simulink model "pid_control"  (R2014a)
settings: Solver=ode45  StartTime=0.0  StopTime=100.0  RelTol=1e-3
libraries: fuzblock x1
settings Model: Creator=Gaea  LastModifiedBy=Gaea

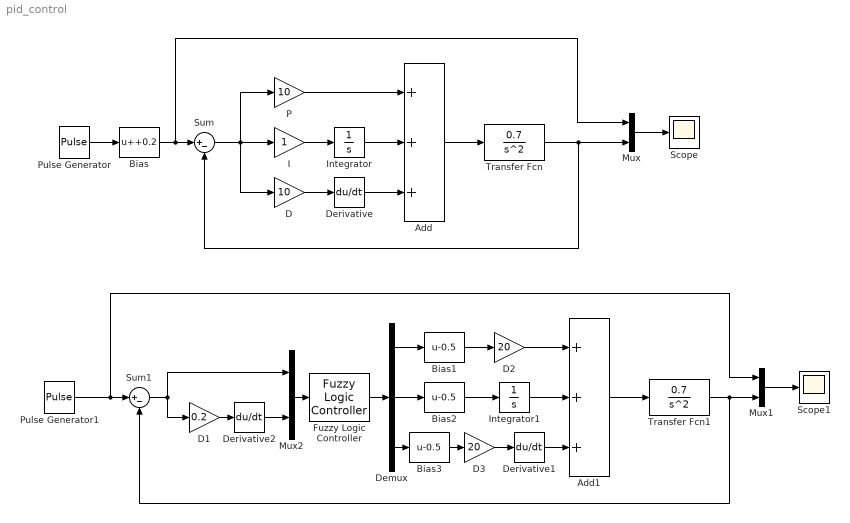
== system pid_control ==
  Add : Sum  Inputs=+++
  Add1 : Sum  Inputs=+++
  Bias : Bias  Bias=+0.2
  Bias1 : Bias  Bias=-0.5
  Bias2 : Bias  Bias=-0.5
  Bias3 : Bias  Bias=-0.5
  D : Gain  Gain=10
  D1 : Gain  Gain=0.2
  D2 : Gain  Gain=20
  D3 : Gain  Gain=20
  Demux : Demux  Outputs=3
  Derivative : Derivative
  Derivative1 : Derivative
  Derivative2 : Derivative
  Fuzzy Logic Controller : fuzblock/Fuzzy Logic  Controller  fis=fc
  I : Gain
  Integrator : Integrator
  Integrator1 : Integrator
  Mux : Mux  Inputs=2
  Mux1 : Mux  Inputs=2
  Mux2 : Mux  Inputs=2
  P : Gain  Gain=10
  Pulse Generator : DiscretePulseGenerator  PulseType=Time based  Amplitude=0.1  Period=20  PulseWidth=50
  Pulse Generator1 : DiscretePulseGenerator  PulseType=Time based  Period=20  PulseWidth=50
  Scope : Scope
  Scope1 : Scope
  Sum : Sum  Inputs=|+-
  Sum1 : Sum  Inputs=|+-
  Transfer Fcn : TransferFcn  Numerator=[0.7]  Denominator=[1 0 0]
  Transfer Fcn1 : TransferFcn  Numerator=[0.7]  Denominator=[1 0 0]
  wires:
  Pulse Generator/1 -> Bias/1
  Transfer Fcn/1 -> Mux/2, Sum/2
  Mux/1 -> Scope/1
  Add/1 -> Transfer Fcn/1
  P/1 -> Add/1
  I/1 -> Integrator/1
  Integrator/1 -> Add/2
  Derivative/1 -> Add/3
  D/1 -> Derivative/1
  Bias/1 -> Mux/1, Sum/1
  Sum/1 -> D/1, P/1, I/1
  Transfer Fcn1/1 -> Mux1/2, Sum1/2
  Mux1/1 -> Scope1/1
  Add1/1 -> Transfer Fcn1/1
  Demux/1 -> Bias1/1
  Demux/2 -> Bias2/1
  Integrator1/1 -> Add1/2
  Derivative1/1 -> Add1/3
  Pulse Generator1/1 -> Mux1/1, Sum1/1
  Mux2/1 -> Fuzzy Logic Controller/1
  Fuzzy Logic Controller/1 -> Demux/1
  Derivative2/1 -> Mux2/2
  Sum1/1 -> D1/1, Mux2/1
  D1/1 -> Derivative2/1
  D2/1 -> Add1/1
  D3/1 -> Derivative1/1
  Bias1/1 -> D2/1
  Bias2/1 -> Integrator1/1
  Demux/3 -> Bias3/1
  Bias3/1 -> D3/1
